simulink model "control_model_working_logic"  (R2025a)
settings: Solver=VariableStepAuto  StartTime=0.0  StopTime=50  RelTol=1e-3
settings Model: Creator=Deepak  LastModifiedBy=Deepak

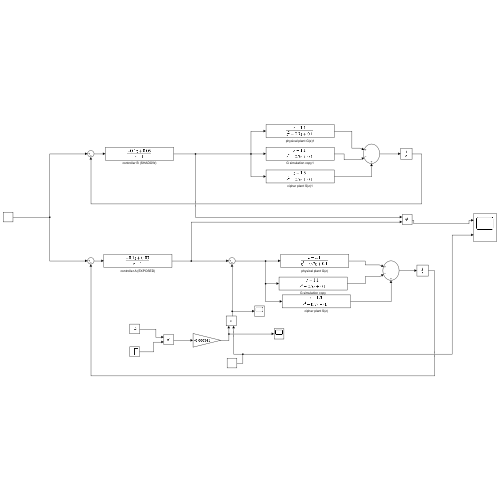
[thumbnail: Simulink's stored preview of the top-level diagram]
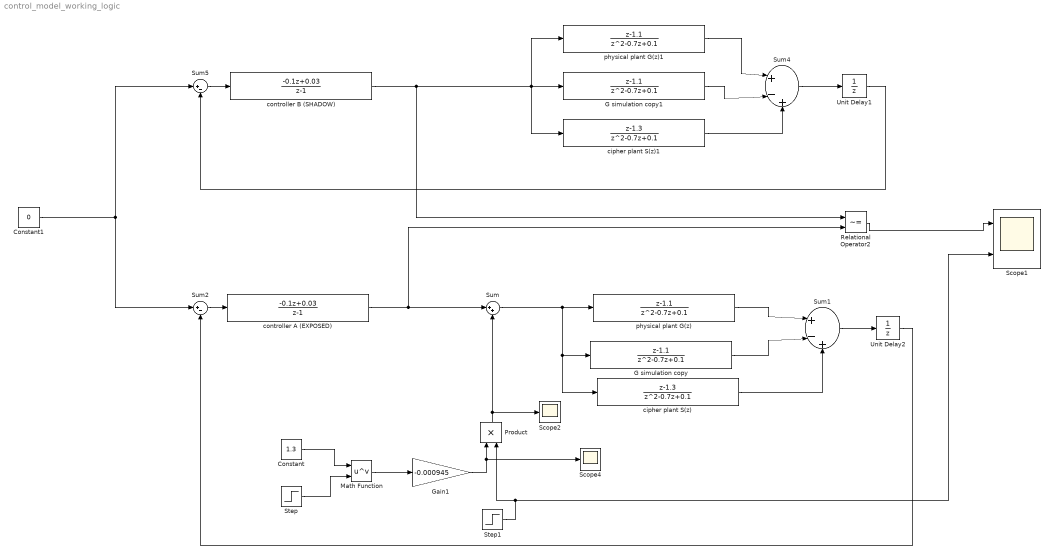
== system control_model_working_logic ==
  Constant : Constant  Value=1.3
  Constant1 : Constant  Value=0
  G simulation copy : DiscreteTransferFcn  Numerator=[1, -1.1]  Denominator=[1, -0.7, 0.1]
  G simulation copy1 : DiscreteTransferFcn  Numerator=[1, -1.1]  Denominator=[1, -0.7, 0.1]
  Gain1 : Gain  Gain=-0.000945
  Math Function : Math  Operator=pow
  Product : Product
  Relational Operator2 : RelationalOperator  Operator=~=  OutDataTypeStr=boolean  RndMeth=Simplest  InputSameDT=off
  Scope1 : Scope  NumInputPorts=2
      settings: ActiveDisplayYMinimum=-0.12499999999999997  ActiveDisplayYMaximum=1.125
  Scope2 : Scope
      settings: ActiveDisplayYMinimum=-0.0014523865668457031  ActiveDisplayYMaximum=0.00041417521831054686  DataLoggingVariableName=ScopeData2
  Scope4 : Scope
      settings: ActiveDisplayYMinimum=-0.0012584907369943834  ActiveDisplayYMaximum=-0.0010066430406295214  DataLoggingVariableName=ScopeData4
  Step : Step  Time=20  SampleTime=1  VectorParams1D=off  ZeroCross=off
  Step1 : Step  Time=20  SampleTime=1  VectorParams1D=off  ZeroCross=off
  Sum : Sum  Inputs=|++
  Sum1 : Sum  Inputs=|+-+
  Sum2 : Sum  Inputs=|+-
  Sum4 : Sum  Inputs=|+-+
  Sum5 : Sum  Inputs=|+-
  Unit Delay1 : UnitDelay  SampleTime=0.001  HasFrameUpgradeWarning=on
  Unit Delay2 : UnitDelay  SampleTime=0.001  HasFrameUpgradeWarning=on
  cipher plant S(z) : DiscreteTransferFcn  Numerator=[1, -1.3]  Denominator=[1, -0.7, 0.1]
  cipher plant S(z)1 : DiscreteTransferFcn  Numerator=[1, -1.3]  Denominator=[1, -0.7, 0.1]  SampleTime=1
  controller A (EXPOSED) : DiscreteTransferFcn  Numerator=[-0.1, 0.03]  Denominator=[1, -1]
  controller B (SHADOW) : DiscreteTransferFcn  Numerator=[-0.1, 0.03]  Denominator=[1, -1]
  physical plant G(z) : DiscreteTransferFcn  Numerator=[1, -1.1]  Denominator=[1, -0.7, 0.1]
  physical plant G(z)1 : DiscreteTransferFcn  Numerator=[1, -1.1]  Denominator=[1, -0.7, 0.1]
  wires:
  Unit Delay1/1 -> Sum5/2
  Math Function/1 -> Gain1/1
  controller B (SHADOW)/1 -> Relational Operator2/1, cipher plant S(z)1/1, G simulation copy1/1, physical plant G(z)1/1
  G simulation copy/1 -> Sum1/2
  Sum/1 -> cipher plant S(z)/1, G simulation copy/1, physical plant G(z)/1
  physical plant G(z)/1 -> Sum1/1
  Sum5/1 -> controller B (SHADOW)/1
  G simulation copy1/1 -> Sum4/2
  Constant1/1 -> Sum5/1, Sum2/1
  Sum1/1 -> Unit Delay2/1
  Step1/1 -> Scope1/2, Product/2
  physical plant G(z)1/1 -> Sum4/1
  Constant/1 -> Math Function/1
  controller A (EXPOSED)/1 -> Relational Operator2/2, Sum/1
  Sum2/1 -> controller A (EXPOSED)/1
  Sum4/1 -> Unit Delay1/1
  Gain1/1 -> Product/1, Scope4/1
  Product/1 -> Sum/2, Scope2/1
  cipher plant S(z)1/1 -> Sum4/3
  Step/1 -> Math Function/2
  cipher plant S(z)/1 -> Sum1/3
  Unit Delay2/1 -> Sum2/2
  Relational Operator2/1 -> Scope1/1
